simulink model "Input_Event"  (R2020b)
settings: Solver=VariableStepAuto  StartTime=0.0  StopTime=10.0  RelTol=1e-3
settings Model: Creator=apple  LastModifiedBy=apple

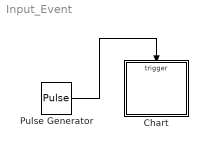
== system Input_Event ==
  Chart : Stateflow chart  TreatAsAtomicUnit=on
  Pulse Generator : DiscretePulseGenerator  PulseType=Time based  Period=10  PulseWidth=5
  wires:
  Pulse Generator/1 -> Chart/Trigger

== stateflow chart Input_Event/Chart ==
  state On
    en:fprintf("Entry_On");
    du:fprintf("During_On");
    ex:fprintf("Exit_On");
  state Off
    en:fprintf("Entry_Off");
    du:fprintf("During_Off");
    ex:fprintf("Exit_Off");
  (default) -> On
  On -> Off : E_one/{send(E_one);}
  Off -> On : E_one
  events: E_one input FUNCTION_CALL_EVENT
